simulink model "Wachadlo_Schemat_1"  (R2018a)
settings: Solver=VariableStepAuto  StartTime=0.0  StopTime=30  RelTol=1e-3
values from neighbouring files (symbols this model uses):
  c = 0.2    [Wah.m]
  g = 10    [Wah.m]
  L = 1    [Wah.m]
  m = 1    [Wah.m]
  T = 1    [Wah.m]
settings Model: Creator=john  LastModifiedBy=john

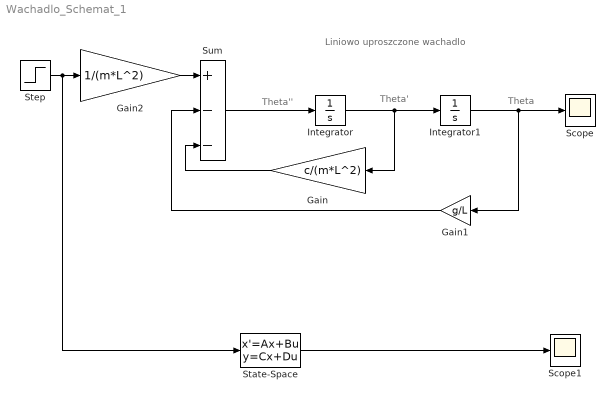
== system Wachadlo_Schemat_1 ==
  note: Liniowo uproszczone wachadlo
  note: Theta''
  note: Theta
  note: Theta'
  Gain : Gain  Gain=c/(m*L^2)
  Gain1 : Gain  Gain=g/L
  Gain2 : Gain  Gain=1/(m*L^2)
  Integrator : Integrator
  Integrator1 : Integrator
  Scope : Scope
  Scope1 : Scope
  State-Space : StateSpace  A=[0,1;-g/L,-c/(m*L^2)]  B=[0;1/(m*L^2)]  C=[1,0]  D=[0]  InitialCondition=0
  Step : Step  After=T  SampleTime=0
  Sum : Sum  Inputs=+--
  wires:
  Integrator/1 -> Gain/1, Integrator1/1
  Integrator1/1 -> Gain1/1, Scope/1
  Sum/1 -> Integrator/1
  Gain/1 -> Sum/3
  Gain1/1 -> Sum/2
  Step/1 -> State-Space/1, Gain2/1
  Gain2/1 -> Sum/1
  State-Space/1 -> Scope1/1
